simulink model "BodyModel_Simulink"  (R2020b)
settings: Solver=ode23tb  StartTime=0.0  StopTime=30  RelTol=1e-3
model workspace (MAT data in the model file):
  A_m = [-1000000  0  0  0  0  0  0  0  0  0  0  0; 0  -1000000  0  0  0  0  0  0  0  0  0  0; 0  0  -1000000  0  0  0  0  0  0  0  0  0; 0  0  0  -1000000  0  0  0  0  0  0  0  0; 0  0  0  0  -1000000  0  0  0  0  0  0  0; 0  0  0  0  0  -1000000  0  0  0  0  0  0; 0  0  0  0  0  0  -1000000  0  0  0  0  0; 0  0  0  0  0  0  0  -1000000  0  0  0  0; 0  0  0  0  0  0  0  0  -1000000  0  0  0; 0  0  0  0  0  0  0  0  0  -1000000  0  0; 0  0  0  0  0  0  0  0  0  0  -1000000  0; 0  0  0  0  0  0  0  0  0  0  0  -1000000]
  B_m = [1000000  0  0  0  0  0  0  0  0  0  0  0; 0  1000000  0  0  0  0  0  0  0  0  0  0; 0  0  1000000  0  0  0  0  0  0  0  0  0; 0  0  0  1000000  0  0  0  0  0  0  0  0; 0  0  0  0  1000000  0  0  0  0  0  0  0; 0  0  0  0  0  1000000  0  0  0  0  0  0; 0  0  0  0  0  0  1000000  0  0  0  0  0; 0  0  0  0  0  0  0  1000000  0  0  0  0; 0  0  0  0  0  0  0  0  1000000  0  0  0; 0  0  0  0  0  0  0  0  0  1000000  0  0; 0  0  0  0  0  0  0  0  0  0  1000000  0; 0  0  0  0  0  0  0  0  0  0  0  1000000]
  C_m = [1  0  0  0  0  0  0  0  0  0  0  0; 0  1  0  0  0  0  0  0  0  0  0  0; 0  0  1  0  0  0  0  0  0  0  0  0; 0  0  0  1  0  0  0  0  0  0  0  0; 0  0  0  0  1  0  0  0  0  0  0  0; 0  0  0  0  0  1  0  0  0  0  0  0; 0  0  0  0  0  0  1  0  0  0  0  0; 0  0  0  0  0  0  0  1  0  0  0  0; 0  0  0  0  0  0  0  0  1  0  0  0; 0  0  0  0  0  0  0  0  0  1  0  0; 0  0  0  0  0  0  0  0  0  0  1  0; 0  0  0  0  0  0  0  0  0  0  0  1]
  D_m = [0  0  0  0  0  0  0  0  0  0  0  0; 0  0  0  0  0  0  0  0  0  0  0  0; 0  0  0  0  0  0  0  0  0  0  0  0; 0  0  0  0  0  0  0  0  0  0  0  0; 0  0  0  0  0  0  0  0  0  0  0  0; 0  0  0  0  0  0  0  0  0  0  0  0; 0  0  0  0  0  0  0  0  0  0  0  0; 0  0  0  0  0  0  0  0  0  0  0  0; 0  0  0  0  0  0  0  0  0  0  0  0; 0  0  0  0  0  0  0  0  0  0  0  0; 0  0  0  0  0  0  0  0  0  0  0  0; 0  0  0  0  0  0  0  0  0  0  0  0]
  K_lqr = [5.00001010272  -4.99939075516  -5  7.78082567543  -7.78909762124  -28.2050033798  34.9965014575  34.8539714107  5.00059906911  8.26036168298  8.18307886119  11.6702457142; 4.99998989726  4.99939075501  -5  7.78080049978  7.7890933152  -28.2050033798  -34.996435735  34.8541161166  -5.00061927225  -8.26033252201  8.18359860677  -11.670303435; -4.99998989957  5.00060917077  -5  -7.78080480918  7.79035830408  -28.2050033798  -34.9838413274  -34.8541818537  4.99940085665  -8.22726404921  -8.18362777058  11.6668224683; -5.00001010041  -5.00060917062  -5  -7.78082136603  -7.79035399804  -28.2050033798  34.9837756048  -34.8539056735  -4.9993806535  8.22723488823  -8.18304969739  -11.6667647475]
  QuadrotorBodyModel_Object : BodyModel (value not decoded)
  u_ss = [1511.25604245; 1511.25604245; 1511.25604245; 1511.25604245]
  x_des = [10; 10; -10; 0; 0; 0; 0; 0; 0; 0; 0; 0]
symbols that are objects in the model workspace (value not decoded): QuadrotorBodyModel_Object
libraries: uavutilslib x1
settings Model: OrderedModelArguments=off  Creator=prenk  LastModifiedBy=renkert2
settings DataIOCC: SaveFormat=Array

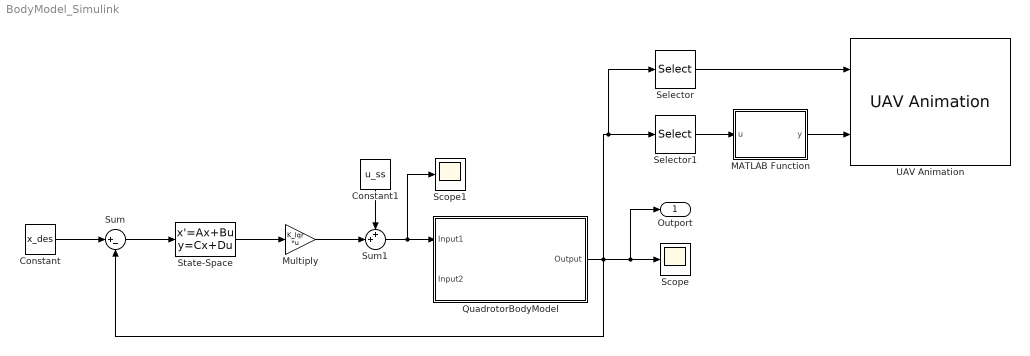
== system BodyModel_Simulink ==
  Constant : Constant  Value=x_des  VectorParams1D=off
  Constant1 : Constant  Value=u_ss  VectorParams1D=off
  MATLAB Function : MATLAB Function  TreatAsAtomicUnit=on
  Multiply : Gain  Gain=K_lqr  Multiplication=Matrix(K*u)
  QuadrotorBodyModel : Subsystem  mask{x_0=[0;0;0;0;0;0;0;0;0;0;0;0]}
  Scope : Scope
  Scope1 : Scope
  Selector : Selector  InputPortWidth=QuadrotorBodyModel_Object.Nx  IndexOptions=Index vector (dialog)  Indices=QuadrotorBodyModel_Object.I.x.p  OutputSizes=1
  Selector1 : Selector  InputPortWidth=QuadrotorBodyModel_Object.Nx  IndexOptions=Index vector (dialog)  Indices=QuadrotorBodyModel_Object.I.x.Theta  OutputSizes=1
  State-Space : StateSpace  A=A_m  B=B_m  C=C_m  D=D_m  InitialCondition=0
  Sum : Sum  Inputs=|+-
  Sum1 : Sum  Inputs=++|
  UAV Animation : uavutilslib/UAV Animation  UAVType=Multirotor  UAVSize=1  InertialZDirection=Down  SampleTime=-1
      settings: SourceProductBaseCode=UV
  Outport : Outport  SignalName=y_out
  wires:
  Constant/1 -> Sum/1
  Constant1/1 -> Sum1/1
  QuadrotorBodyModel/1(Output) -> Sum/2, Outport/1, Scope/1, Selector1/1, Selector/1
  Sum1/1 -> Scope1/1, QuadrotorBodyModel/1(Input1)
  Multiply/1 -> Sum1/2
  Sum/1 -> State-Space/1
  State-Space/1 -> Multiply/1
  Selector/1 -> UAV Animation/1
  Selector1/1 -> MATLAB Function/1(u)
  MATLAB Function/1(y) -> UAV Animation/2

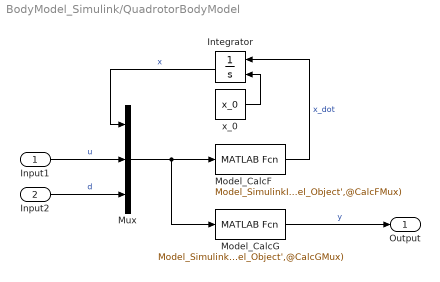
== system BodyModel_Simulink/QuadrotorBodyModel ==
  Input1 : Inport  PortDimensions=[QuadrotorBodyModel_Object.Nu,1]
  Input2 : Inport  Port=2
  Integrator : Integrator  InitialConditionSource=external
  Model_CalcF : MATLABFcn  MATLABFcn=Model_SimulinkInterpretedFunction(u,'BodyModel_Simulink','QuadrotorBodyModel_Object',@CalcFMux)  OutputDimensions=QuadrotorBodyModel_Object.Nx
  Model_CalcG : MATLABFcn  MATLABFcn=Model_SimulinkInterpretedFunction(u,'BodyModel_Simulink','QuadrotorBodyModel_Object',@CalcGMux)  OutputDimensions=QuadrotorBodyModel_Object.Ny
  Mux : Mux  Inputs=3
  x_0 : Constant  Value=x_0  VectorParams1D=off
  Output : Outport
  wires:
  Model_CalcF/1 -> Integrator/1  "x_dot"
  Input1/1 -> Mux/2  "u"
  Model_CalcG/1 -> Output/1  "y"
  x_0/1 -> Integrator/2
  Input2/1 -> Mux/3  "d"
  Integrator/1 -> Mux/1  "x"
  Mux/1 -> Model_CalcG/1, Model_CalcF/1

== matlab function BodyModel_Simulink/MATLAB Function ==
  data: u input; y output
function y = eul2quatMF(u)
    y = eul2quat([1 -1 1].*fliplr(u'),'ZYX');
end
